simulink model "nn"  (R2023a)
settings: Solver=VariableStepAuto  StartTime=0.0  StopTime=10.0  RelTol=1e-3
libraries: neural x122
(part 1 of 5)
settings Model: Creator=wcheng2014  LastModifiedBy=wcheng2014

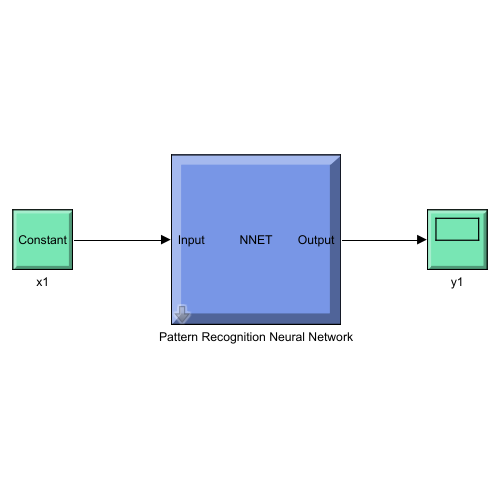
[thumbnail: Simulink's stored preview of the top-level diagram]
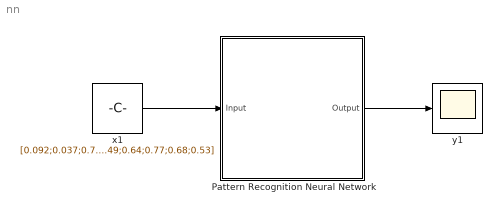
== system nn ==
  Pattern Recognition Neural Network : Subsystem
      mask help: Pattern Recognition Neural Network
      mask Display: e = 0.06;c1 = [120 150 230]/255;c2 = ([120 150 230]+0)/383;c3 = ([120 150 230]+128)/383;patch([0 1 1 0],[0 0 1 1],c1);patch([0 1 1 1-e 1-e 0+e],[0 0 1 1-e 0+e 0+e],c2);patch([0 0 1 1-e 0+e 0+e],[0 1 1 1-e 1-e 0+e],c3);plot([0 1 1 0 0],[0 0 1 1 0]);fprintf('NNET');port_label('input',1,' Input');port_label('output',1,'Output ');
  x1 : Constant  Value=[0.092;0.037;0.78;0.038;0.97;0.48;0.48;0.37;0.98;0.66;0.58;0.29;0.96;0.22;0.87;0.29;0.71;0.97;0.96;0.49;0.64;0.77;0.68;0.53]  SampleTime=1
      mask Display: e = 0.06;c1 = [120 230 180]/255;c2 = ([120 230 180]+0)/(256+128);c3 = ([120 230 180]+128)/(256+128);patch([0 1 1 0],[0 0 1 1],c1);patch([0 1 1 1-e 1-e 0+e],[0 0 1 1-e 0+e 0+e],c2);patch([0 0 1 1-e 0+e 0+e],[0 1 1 1-e 1-e 0+e],c3);plot([0 1 1 0 0],[0 0 1 1 0]);disp('Constant');
  y1 : Scope
      mask Display: e = 0.06;c1 = [120 230 180]/255;c2 = ([120 230 180]+0)/(256+128);c3 = ([120 230 180]+128)/(256+128);patch([0 1 1 0],[0 0 1 1],c1);patch([0 1 1 1-e 1-e 0+e],[0 0 1 1-e 0+e 0+e],c2);patch([0 0 1 1-e 0+e 0+e],[0 1 1 1-e 1-e 0+e],c3);plot([0 1 1 0 0],[0 0 1 1 0]);plot([0.15 0.85 0.85 0.15 0.15],[0.5 0.5 0.85 0.85 0.5]);
  wires:
  x1/1 -> Pattern Recognition Neural Network/1(Input)
  Pattern Recognition Neural Network/1(Output) -> y1/1

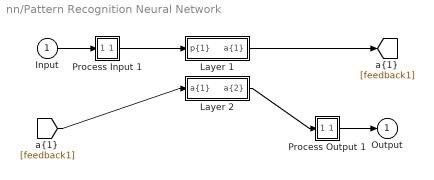
== system nn/Pattern Recognition Neural Network ==
  Input : Inport  PortDimensions=24
      mask Display: e = 0.06;c1 = [120 230 180]/255;c2 = ([120 230 180]+0)/(256+128);c3 = ([120 230 180]+128)/(256+128);patch([0 1 1 0],[0 0 1 1],c1);patch([0 1 1 1-e 1-e 0+e],[0 0 1 1-e 0+e 0+e],c2);patch([0 0 1 1-e 0+e 0+e],[0 1 1 1-e 1-e 0+e],c3);plot([0 1 1 0 0],[0 0 1 1 0]);
  Layer 1 : Subsystem
      mask Display: e = 0.06;c1 = [120 150 230]/255;c2 = ([120 150 230]+0)/383;c3 = ([120 150 230]+128)/383;patch([0 1 1 0],[0 0 1 1],c1);patch([0 1 1 1-e 1-e 0+e],[0 0 1 1-e 0+e 0+e],c2);patch([0 0 1 1-e 0+e 0+e],[0 1 1 1-e 1-e 0+e],c3);plot([0 1 1 0 0],[0 0 1 1 0]);
  Layer 2 : Subsystem
      mask Display: e = 0.06;c1 = [120 150 230]/255;c2 = ([120 150 230]+0)/383;c3 = ([120 150 230]+128)/383;patch([0 1 1 0],[0 0 1 1],c1);patch([0 1 1 1-e 1-e 0+e],[0 0 1 1-e 0+e 0+e],c2);patch([0 0 1 1-e 0+e 0+e],[0 1 1 1-e 1-e 0+e],c3);plot([0 1 1 0 0],[0 0 1 1 0]);
  Process Input 1 : Subsystem
      mask Display: e = 0.06;c1 = [120 150 230]/255;c2 = ([120 150 230]+0)/383;c3 = ([120 150 230]+128)/383;patch([0 1 1 0],[0 0 1 1],c1);patch([0 1 1 1-e 1-e 0+e],[0 0 1 1-e 0+e 0+e],c2);patch([0 0 1 1-e 0+e 0+e],[0 1 1 1-e 1-e 0+e],c3);plot([0 1 1 0 0],[0 0 1 1 0]);
  Process Output 1 : Subsystem
      mask Display: e = 0.06;c1 = [120 150 230]/255;c2 = ([120 150 230]+0)/383;c3 = ([120 150 230]+128)/383;patch([0 1 1 0],[0 0 1 1],c1);patch([0 1 1 1-e 1-e 0+e],[0 0 1 1-e 0+e 0+e],c2);patch([0 0 1 1-e 0+e 0+e],[0 1 1 1-e 1-e 0+e],c3);plot([0 1 1 0 0],[0 0 1 1 0]);
  Output : Outport  InitialOutput=[0;0;0;0;0;0;0;0;0;0;0;0;0;0;0;0;0;0;0]
      mask Display: e = 0.06;c1 = [120 230 180]/255;c2 = ([120 230 180]+0)/(256+128);c3 = ([120 230 180]+128)/(256+128);patch([0 1 1 0],[0 0 1 1],c1);patch([0 1 1 1-e 1-e 0+e],[0 0 1 1-e 0+e 0+e],c2);patch([0 0 1 1-e 0+e 0+e],[0 1 1 1-e 1-e 0+e],c3);plot([0 1 1 0 0],[0 0 1 1 0]);
  wires:
  Input/1 -> Process Input 1/1(x)
  Process Output 1/1(y) -> Output/1
  Process Input 1/1(p) -> Layer 1/1("p{1}")
  Layer 1/1("a{1}") -> [feedback1]
  [feedback1] -> Layer 2/1("a{1} ")
  Layer 2/1("a{2}") -> Process Output 1/1(a)

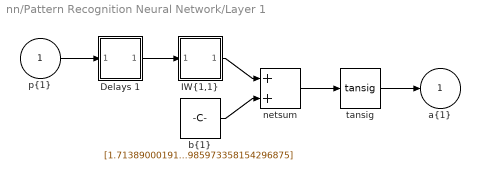
== system nn/Pattern Recognition Neural Network/Layer 1 ==
  "p{1}" : Inport  PortDimensions=24
      mask Display: e = 0.06;c1 = [120 230 180]/255;c2 = ([120 230 180]+0)/(256+128);c3 = ([120 230 180]+128)/(256+128);patch([0 1 1 0],[0 0 1 1],c1);patch([0 1 1 1-e 1-e 0+e],[0 0 1 1-e 0+e 0+e],c2);patch([0 0 1 1-e 0+e 0+e],[0 1 1 1-e 1-e 0+e],c3);plot([0 1 1 0 0],[0 0 1 1 0]);
  Delays 1 : Subsystem
      mask Display: e = 0.06;c1 = [120 150 230]/255;c2 = ([120 150 230]+0)/383;c3 = ([120 150 230]+128)/383;patch([0 1 1 0],[0 0 1 1],c1);patch([0 1 1 1-e 1-e 0+e],[0 0 1 1-e 0+e 0+e],c2);patch([0 0 1 1-e 0+e 0+e],[0 1 1 1-e 1-e 0+e],c3);plot([0 1 1 0 0],[0 0 1 1 0]);disp('0');
  "IW{1,1}" : Subsystem
      mask Display: e = 0.06;c1 = [120 150 230]/255;c2 = ([120 150 230]+0)/383;c3 = ([120 150 230]+128)/383;patch([0 1 1 0],[0 0 1 1],c1);patch([0 1 1 1-e 1-e 0+e],[0 0 1 1-e 0+e 0+e],c2);patch([0 0 1 1-e 0+e 0+e],[0 1 1 1-e 1-e 0+e],c3);plot([0 1 1 0 0],[0 0 1 1 0]);disp('W');
  "b{1}" : Constant  Value=[1.7138900019148344266994854478980414569377899169921875;-2.471374304738606308973203340428881347179412841796875;-1.835709839130736487078365826164372265338897705078125;1.825216660047917827114360989071428775787353515625;-1.4098518847714289758954464559792540967464447021484375;1.1210163424962036327059422546881251037120819091796875;-1.2088364371651632023230149570736102759838104248046875;-1.79596080897342336157862519030459225177764892578125;-1.2289475291366616094279606841155327856540679931640625;1.4783375225635475569418986196978949010372161865234375;-1.4511034566389271471820165970711968839168548583984375;1.095438631047267907803188791149295866489410400390625;-0.4288344387461024975749523946433328092098236083984375;0.62791342573735631216180763658485375344753265380859375;1.954829433629265533767238594009540975093841552734375;1.3978577326526941959627947653643786907196044921875;-0.81115599899778556558516129371128045022487640380859375;-1.335980008320762468798648114898242056369781494140625;-1.4565276871204624331568311390583403408527374267578125;1.12018535982015254859334163484163582324981689453125;-0.77538230543580877185405597629141993820667266845703125;1.21776958986870287304782323190011084079742431640625;0.7889652053242743878769260845729149878025054931640625;1.1195232509345627303076753378263674676418304443359375;0.284652545538766954535958575434051454067230224609375;-0.0025978070374918309747014344424087539664469659328460693359375;0.58932675347992413694697688697488047182559967041015625;-0.181908652326444097990787440721760503947734832763671875;0.0653788251888795246546948192190029658377170562744140625;1.551212449575257945610928800306282937526702880859375;-0.5548614974805887722908437353908084332942962646484375;-0.1601364401496910006006402227285434491932392120361328125;-1.059116928434203686038017622195184230804443359375;1.1558933761582093069364418624900281429290771484375;0.35569956179120854056208145266282372176647186279296875;0.96511581635036858273224424920044839382171630859375;-0.157909106825796730078081964165903627872467041015625;1.4413185664313015177384613707545213401317596435546875;-0.46101273158599453960704295241157524287700653076171875;0.349128375544600577651266348766512237489223480224609375;-0.452342664744146805144708878287929110229015350341796875;-0.05670793079071610731656249981824657879769802093505859375;-0.07720341369440160417259022551661473698914051055908203125;-0.395579924584184450253587783663533627986907958984375;0.11805002410444066784922512169941910542547702789306640625;-0.77318354413052270412975985891534946858882904052734375;0.62381483552428651506716050789691507816314697265625;-0.0174314996309005466879060719520566635765135288238525390625;0.30647979703073635615595549097633920609951019287109375;0.07113809751572448825118755166840855963528156280517578125;-0.3380149976659716504201469433610327541828155517578125;-0.9353842060813548631159619617392309010028839111328125;-0.1639802381044829504563864475130685605108737945556640625;-0.82537878200821135354914304116391576826572418212890625;0.311038194959184000065732789153116755187511444091796875;-0.5811696960035543924050216446630656719207763671875;-1.1522248622329327449875790989608503878116607666015625;0.74642138572876015611967659424408338963985443115234375;-0.98043670102208679839606020323117263615131378173828125;0.372256236870946610739707693937816657125949859619140625;0.3621700554911548852743408133392222225666046142578125;0.353949146537022585334852919913828372955322265625;-1.187579092949061720929648799938149750232696533203125;0.41113461021127883920911472159787081182003021240234375;-0.34386793596550291329805304485489614307880401611328125;-1.338801216649933234492664269055239856243133544921875;0.87009942390120087463145637229899875819683074951171875;-0.358965589519839645138432615567580796778202056884765625;-0.06876750624335149775223641199772828258574008941650390625;-0.59964798689309450896445241596666164696216583251953125;-0.56481919299235905373990362932090647518634796142578125 ...(+1608 chars)]
      mask Display: e = 0.06;c1 = [120 150 230]/255;c2 = ([120 150 230]+0)/383;c3 = ([120 150 230]+128)/383;patch([0 1 1 0],[0 0 1 1],c1);patch([0 1 1 1-e 1-e 0+e],[0 0 1 1-e 0+e 0+e],c2);patch([0 0 1 1-e 0+e 0+e],[0 1 1 1-e 1-e 0+e],c3);plot([0 1 1 0 0],[0 0 1 1 0]);disp('b');
  netsum : Sum  Inputs=2  InputSameDT=on  SaturateOnIntegerOverflow=on  OutDataTypeStr=Inherit: Same as first input
      mask Display: e = 0.06;c1 = [120 150 230]/255;c2 = ([120 150 230]+0)/383;c3 = ([120 150 230]+128)/383;patch([0 1 1 0],[0 0 1 1],c1);patch([0 1 1 1-e 1-e 0+e],[0 0 1 1-e 0+e 0+e],c2);patch([0 0 1 1-e 0+e 0+e],[0 1 1 1-e 1-e 0+e],c3);plot([0 1 1 0 0],[0 0 1 1 0]);disp('+');
  tansig : neural/Transfer Functions/tansig
  "a{1}" : Outport  InitialOutput=[0;0;0;0;0;0;0;0;0;0;0;0;0;0;0;0;0;0;0;0;0;0;0;0;0;0;0;0;0;0;0;0;0;0;0;0;0;0;0;0;0;0;0;0;0;0;0;0;0;0;0;0;0;0;0;0;0;0;0;0;0;0;0;0;0;0;0;0;0;0;0;0;0;0;0;0;0;0;0;0;0;0;0;0;0;0;0;0;0;0;0;0;0;0;0;0;0;0;0;0]
      mask Display: e = 0.06;c1 = [120 230 180]/255;c2 = ([120 230 180]+0)/(256+128);c3 = ([120 230 180]+128)/(256+128);patch([0 1 1 0],[0 0 1 1],c1);patch([0 1 1 1-e 1-e 0+e],[0 0 1 1-e 0+e 0+e],c2);patch([0 0 1 1-e 0+e 0+e],[0 1 1 1-e 1-e 0+e],c3);plot([0 1 1 0 0],[0 0 1 1 0]);
  wires:
  "p{1}"/1 -> Delays 1/1("p{1}")
  Delays 1/1("pd{1,1}") -> "IW{1,1}"/1("pd{1,1}")
  "IW{1,1}"/1("iz{1,1}") -> netsum/1
  "b{1}"/1 -> netsum/2
  netsum/1 -> tansig/1
  tansig/1 -> "a{1}"/1

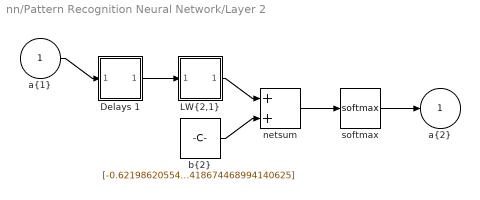
== system nn/Pattern Recognition Neural Network/Layer 2 ==
  "a{1} " : Inport  PortDimensions=100
      mask Display: e = 0.06;c1 = [120 230 180]/255;c2 = ([120 230 180]+0)/(256+128);c3 = ([120 230 180]+128)/(256+128);patch([0 1 1 0],[0 0 1 1],c1);patch([0 1 1 1-e 1-e 0+e],[0 0 1 1-e 0+e 0+e],c2);patch([0 0 1 1-e 0+e 0+e],[0 1 1 1-e 1-e 0+e],c3);plot([0 1 1 0 0],[0 0 1 1 0]);
  Delays 1 : Subsystem
      mask Display: e = 0.06;c1 = [120 150 230]/255;c2 = ([120 150 230]+0)/383;c3 = ([120 150 230]+128)/383;patch([0 1 1 0],[0 0 1 1],c1);patch([0 1 1 1-e 1-e 0+e],[0 0 1 1-e 0+e 0+e],c2);patch([0 0 1 1-e 0+e 0+e],[0 1 1 1-e 1-e 0+e],c3);plot([0 1 1 0 0],[0 0 1 1 0]);disp('0');
  "LW{2,1}" : Subsystem
      mask Display: e = 0.06;c1 = [120 150 230]/255;c2 = ([120 150 230]+0)/383;c3 = ([120 150 230]+128)/383;patch([0 1 1 0],[0 0 1 1],c1);patch([0 1 1 1-e 1-e 0+e],[0 0 1 1-e 0+e 0+e],c2);patch([0 0 1 1-e 0+e 0+e],[0 1 1 1-e 1-e 0+e],c3);plot([0 1 1 0 0],[0 0 1 1 0]);disp('W');
  "b{2}" : Constant  Value=[-0.62198620554685468686528793114121071994304656982421875;-0.8980764497228601594969177313032560050487518310546875;-0.614149746349200054140737847774289548397064208984375;-0.44364989261659892871847432616050355136394500732421875;0.30911898031798556996108118255506269633769989013671875;-0.89433521870556165200838449891307391226291656494140625;-0.01524816871858734879108254745005979202687740325927734375;0.441262563565768317630499950610101222991943359375;0.218866592030768802867868316752719692885875701904296875;-0.72816702293418245073297612179885618388652801513671875;0.288488408320161593412223055565846152603626251220703125;-0.380423582403461024714630411835969425737857818603515625;-0.8961841348605308343877595689264126121997833251953125;-0.2074966259284465042167511228399234823882579803466796875;0.54830881691580579673228612591628916561603546142578125;1.1090694711082804690960301741142757236957550048828125;0.1380702072046389450310499569241073913872241973876953125;-0.806215084574514850856985503924079239368438720703125;0.0996990433865324876538949183668592013418674468994140625]
      mask Display: e = 0.06;c1 = [120 150 230]/255;c2 = ([120 150 230]+0)/383;c3 = ([120 150 230]+128)/383;patch([0 1 1 0],[0 0 1 1],c1);patch([0 1 1 1-e 1-e 0+e],[0 0 1 1-e 0+e 0+e],c2);patch([0 0 1 1-e 0+e 0+e],[0 1 1 1-e 1-e 0+e],c3);plot([0 1 1 0 0],[0 0 1 1 0]);disp('b');
  netsum : Sum  Inputs=2  InputSameDT=on  SaturateOnIntegerOverflow=on  OutDataTypeStr=Inherit: Same as first input
      mask Display: e = 0.06;c1 = [120 150 230]/255;c2 = ([120 150 230]+0)/383;c3 = ([120 150 230]+128)/383;patch([0 1 1 0],[0 0 1 1],c1);patch([0 1 1 1-e 1-e 0+e],[0 0 1 1-e 0+e 0+e],c2);patch([0 0 1 1-e 0+e 0+e],[0 1 1 1-e 1-e 0+e],c3);plot([0 1 1 0 0],[0 0 1 1 0]);disp('+');
  softmax : neural/Transfer Functions/softmax
  "a{2}" : Outport  InitialOutput=[0;0;0;0;0;0;0;0;0;0;0;0;0;0;0;0;0;0;0]
      mask Display: e = 0.06;c1 = [120 230 180]/255;c2 = ([120 230 180]+0)/(256+128);c3 = ([120 230 180]+128)/(256+128);patch([0 1 1 0],[0 0 1 1],c1);patch([0 1 1 1-e 1-e 0+e],[0 0 1 1-e 0+e 0+e],c2);patch([0 0 1 1-e 0+e 0+e],[0 1 1 1-e 1-e 0+e],c3);plot([0 1 1 0 0],[0 0 1 1 0]);
  wires:
  "a{1} "/1 -> Delays 1/1("p{2}")
  Delays 1/1("pd{2,1}") -> "LW{2,1}"/1("ad{2,1}")
  "LW{2,1}"/1("lz{2,1}") -> netsum/1
  "b{2}"/1 -> netsum/2
  netsum/1 -> softmax/1
  softmax/1 -> "a{2}"/1

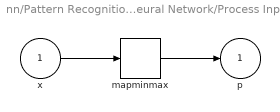
== system nn/Pattern Recognition Neural Network/Process Input 1 ==
  x : Inport  PortDimensions=24
      mask Display: e = 0.06;c1 = [120 230 180]/255;c2 = ([120 230 180]+0)/(256+128);c3 = ([120 230 180]+128)/(256+128);patch([0 1 1 0],[0 0 1 1],c1);patch([0 1 1 1-e 1-e 0+e],[0 0 1 1-e 0+e 0+e],c2);patch([0 0 1 1-e 0+e 0+e],[0 1 1 1-e 1-e 0+e],c3);plot([0 1 1 0 0],[0 0 1 1 0]);
  mapminmax : neural/Processing Functions/mapminmax  xmin=[-0.00177907544467714728853025007993;-0.000396249408619375742546253604814;-0.000665517026475992423684147070162;-0.00283569538946126797895885829348;-0.00144994844225543317861593095586;-0.000543779668398691740094363922253;-0.000342578604035637113156553823501;-0.000509106830160366286008866154589;-0.00158720068081841247931151883677;-0.00047475779492822667293694394175;-0.000849392465379406047532029333524;-0.00048564489986313574831910955254;-0.000466185604408586584668228169903;-0.00028681256207852001693936472293;-0.000590902266625725758331100223586;-0.000379140335352357027431935421191;-0.000241835689680502952114693471231;-0.0010076962340961337361022742698;-0.000451226024864137542635944555514;-0.000362255152537738212004114757292;-0.00060435113556644992627298051957;-0.000470729508835088239493416040204;-0.00145266642471186813168060325552;-0.000695440717817241704779007704929]  xmax=[0.015912572746501041365263517946;0.0100805765840283889644979353761;0.00993380031723223311246329103597;0.00834512271652343429195752833039;0.00654012987079477525753645750228;0.00726238112196719853841386793647;0.00794493787876282553384044149425;0.00737584844500016600932212895714;0.00663887503445259596901451004669;0.00556033159125401965638957335614;0.00616471179048794226673635421321;0.00521187683950286029244125529658;0.00381682131647664846241241320968;0.00389300714770346445448012673296;0.00422909328134934980880643706769;0.00402248649784242573446135793347;0.00559789598245963304634642554447;0.00422840492513021359854974434711;0.00533719235494345412007533013821;0.00626496965036249520153432968073;0.00363632903513355643099203007296;0.00315764470316315382092398067471;0.00318622464416140616094708093442;0.00141976561595580363928092992865]  ymin=-1  ymax=1
  p : Outport  PortDimensions=24
      mask Display: e = 0.06;c1 = [120 230 180]/255;c2 = ([120 230 180]+0)/(256+128);c3 = ([120 230 180]+128)/(256+128);patch([0 1 1 0],[0 0 1 1],c1);patch([0 1 1 1-e 1-e 0+e],[0 0 1 1-e 0+e 0+e],c2);patch([0 0 1 1-e 0+e 0+e],[0 1 1 1-e 1-e 0+e],c3);plot([0 1 1 0 0],[0 0 1 1 0]);
  wires:
  x/1 -> mapminmax/1
  mapminmax/1 -> p/1

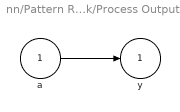
== system nn/Pattern Recognition Neural Network/Process Output 1 ==
  a : Inport  PortDimensions=19
      mask Display: e = 0.06;c1 = [120 230 180]/255;c2 = ([120 230 180]+0)/(256+128);c3 = ([120 230 180]+128)/(256+128);patch([0 1 1 0],[0 0 1 1],c1);patch([0 1 1 1-e 1-e 0+e],[0 0 1 1-e 0+e 0+e],c2);patch([0 0 1 1-e 0+e 0+e],[0 1 1 1-e 1-e 0+e],c3);plot([0 1 1 0 0],[0 0 1 1 0]);
  y : Outport  PortDimensions=19
      mask Display: e = 0.06;c1 = [120 230 180]/255;c2 = ([120 230 180]+0)/(256+128);c3 = ([120 230 180]+128)/(256+128);patch([0 1 1 0],[0 0 1 1],c1);patch([0 1 1 1-e 1-e 0+e],[0 0 1 1-e 0+e 0+e],c2);patch([0 0 1 1-e 0+e 0+e],[0 1 1 1-e 1-e 0+e],c3);plot([0 1 1 0 0],[0 0 1 1 0]);
  wires:
  a/1 -> y/1

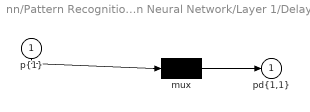
== system nn/Pattern Recognition Neural Network/Layer 1/Delays 1 ==
  "p{1}" : Inport  PortDimensions=24
      mask Display: e = 0.06;c1 = [120 230 180]/255;c2 = ([120 230 180]+0)/(256+128);c3 = ([120 230 180]+128)/(256+128);patch([0 1 1 0],[0 0 1 1],c1);patch([0 1 1 1-e 1-e 0+e],[0 0 1 1-e 0+e 0+e],c2);patch([0 0 1 1-e 0+e 0+e],[0 1 1 1-e 1-e 0+e],c3);plot([0 1 1 0 0],[0 0 1 1 0]);
  mux : Mux  Inputs=1
      mask Display: e = 0.06;c1 = [120 150 230]/255;c2 = ([120 150 230]+0)/383;c3 = ([120 150 230]+128)/383;patch([0 1 1 0],[0 0 1 1],c1);patch([0 1 1 1-e 1-e 0+e],[0 0 1 1-e 0+e 0+e],c2);patch([0 0 1 1-e 0+e 0+e],[0 1 1 1-e 1-e 0+e],c3);plot([0 1 1 0 0],[0 0 1 1 0]);disp('Mux')
  "pd{1,1}" : Outport
      mask Display: e = 0.06;c1 = [120 230 180]/255;c2 = ([120 230 180]+0)/(256+128);c3 = ([120 230 180]+128)/(256+128);patch([0 1 1 0],[0 0 1 1],c1);patch([0 1 1 1-e 1-e 0+e],[0 0 1 1-e 0+e 0+e],c2);patch([0 0 1 1-e 0+e 0+e],[0 1 1 1-e 1-e 0+e],c3);plot([0 1 1 0 0],[0 0 1 1 0]);
  wires:
  "p{1}"/1 -> mux/1
  mux/1 -> "pd{1,1}"/1
